simulink subsystem "Lorenz"  (R2021b)
settings: Solver=VariableStepAuto  StartTime=0.0  StopTime=10.0  RelTol=1e-3
settings Model: Creator=karti  LastModifiedBy=karti

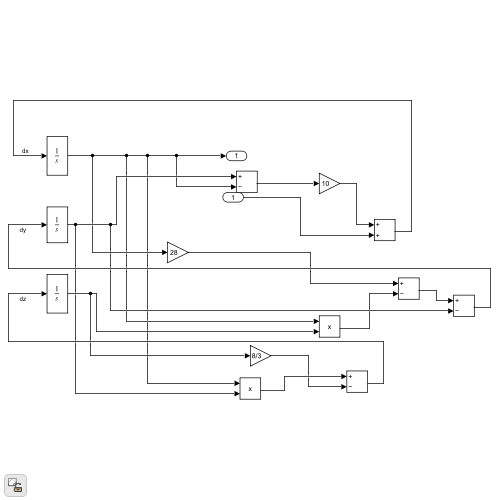
[thumbnail: Simulink's stored preview of the top-level diagram]
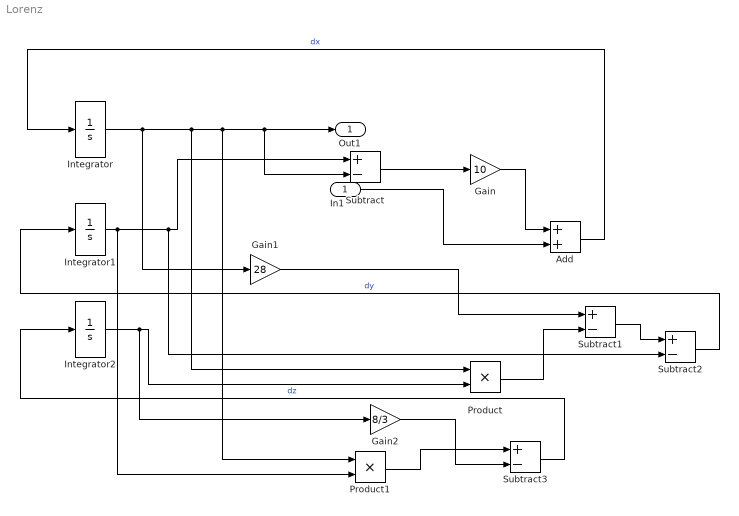
== system Lorenz ==
  In1 : Inport
  Add : Sum
  Gain : Gain  Gain=10
  Gain1 : Gain  Gain=28
  Gain2 : Gain  Gain=8/3
  Integrator : Integrator
  Integrator1 : Integrator  InitialCondition=1
  Integrator2 : Integrator  InitialCondition=20
  Product : Product
  Product1 : Product
  Subtract{,1..3} (4 alike) : Sum  Inputs=+-
  Out1 : Outport
  wires:
  Gain/1 -> Add/1
  Add/1 -> Integrator/1  "dx"
  Subtract2/1 -> Integrator1/1  "dy"
  Integrator1/1 -> Subtract/1, Subtract2/2, Product1/2
  Product/1 -> Subtract1/2
  Integrator/1 -> Subtract/2, Out1/1, Product1/1, Product/1, Gain1/1
  Subtract1/1 -> Subtract2/1
  Subtract/1 -> Gain/1
  Subtract3/1 -> Integrator2/1  "dz"
  Integrator2/1 -> Product/2, Gain2/1
  Product1/1 -> Subtract3/1
  Gain1/1 -> Subtract1/1
  Gain2/1 -> Subtract3/2
  In1/1 -> Add/2
